simulink model "SpeedandTorqueModeComponent"  (R2026a)
settings: Solver=FixedStepDiscrete
settings Model: DataDictionary=TractionEmotorSoftwareArchInterfaceData.sldd  Creator=dakaihu  LastModifiedBy=dakaihu

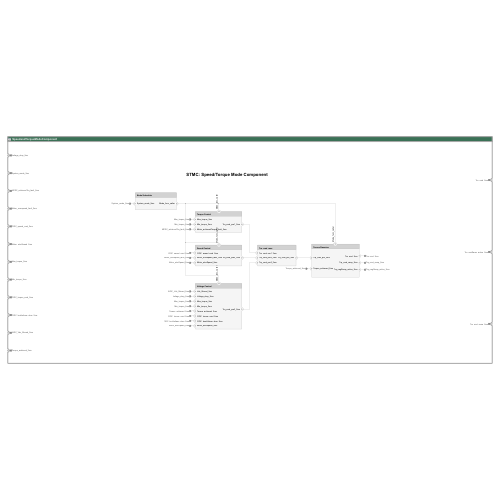
[thumbnail: Simulink's stored preview of the top-level diagram]
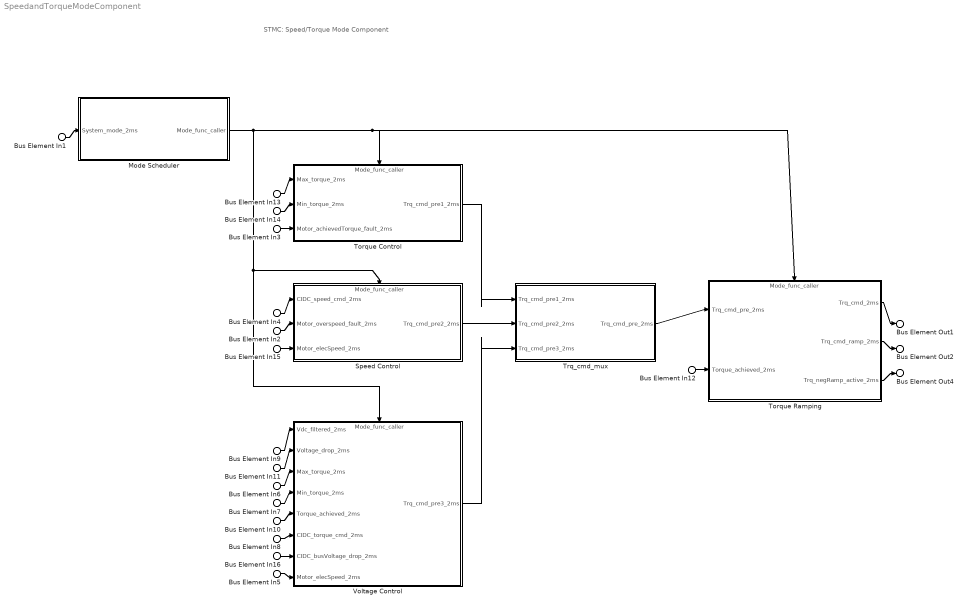
== system SpeedandTorqueModeComponent ==
  note: STMC: Speed/Torque Mode Component
  Bus Element In11 : Inport  PortName=Voltage_drop_2ms
  Bus Element In1 : Inport  Port=2  PortName=System_mode_2ms
  Bus Element In3 : Inport  Port=3  PortName=MFDC_achievedTrq_fault_2ms
  Bus Element In2 : Inport  Port=4  PortName=Motor_overspeed_fault_2ms
  Bus Element In4 : Inport  Port=5  PortName=CIDC_speed_cmd_2ms
  Bus Element In5 : Inport  Port=6  PortName=Motor_elecSpeed_2ms
  Bus Element In15 : Inport  Port=6  PortName=Motor_elecSpeed_2ms
  Bus Element In6 : Inport  Port=7  PortName=Max_torque_2ms
  Bus Element In13 : Inport  Port=7  PortName=Max_torque_2ms
  Bus Element In7 : Inport  Port=8  PortName=Min_torque_2ms
  Bus Element In14 : Inport  Port=8  PortName=Min_torque_2ms
  Bus Element In8 : Inport  Port=9  PortName=CIDC_torque_cmd_2ms
  Bus Element In16 : Inport  Port=10  PortName=CIDC_busVoltage_drop_2ms
  Bus Element In9 : Inport  Port=11  PortName=IHDC_Vdc_filtered_2ms
  Bus Element In10 : Inport  Port=12  PortName=Torque_achieved_2ms
  Bus Element In12 : Inport  Port=12  PortName=Torque_achieved_2ms
  Mode Scheduler : Subsystem
      settings: PortSchema="{\"entries\":[{\"content\":{\"headerSize\":26,\"margin\":15,\"minimumSpacing\":25,\"sides\":[{\"content\":{\"connectorIds\":[\"In1\"]},\"type\":\"ConnectorPlacement.EquallySpacedRectSide\",\"uuid\":\"b2f30fca-3d8e-46ee-af1d-282b22b9b844\"},{\"content\":{\"connectorIds\":[\"Out1\"],\"side\":\"RIGHT\"},\"type\":\"ConnectorPlacement.EquallySpacedRectSide\",\"uuid\":\"2d7d706d-eac4-4c73-84e8-2a36a393a616\"},{\"content\":{\"connectorIds\":[],\"side\":\"TOP\"},\"type\":\"ConnectorPlacement.EquallySpacedRectSide\",\"uuid\":\"b52ae510-b7cc-4ed0-8d34-4a095deae41b\"}]},\"type\":\"ConnectorPlacement.EquallySpacedConnector\",\"uuid\":\"1257e7cc-1858-4bc4-ab05-7b00060cf0d5\"}],\"packageUris\":[\"http://schema.mathworks.com/mf0/Connector/R2020b\"],\"version\":\"1.0\"}"
  Speed Control : Subsystem
      settings: PortSchema="{\"entries\":[{\"content\":{\"headerSize\":26,\"margin\":15,\"minimumSpacing\":25,\"sides\":[{\"content\":{\"connectorIds\":[\"In1\",\"In2\",\"In3\"]},\"type\":\"ConnectorPlacement.EquallySpacedRectSide\",\"uuid\":\"b2f30fca-3d8e-46ee-af1d-282b22b9b844\"},{\"content\":{\"connectorIds\":[\"Out1\"],\"side\":\"RIGHT\"},\"type\":\"ConnectorPlacement.EquallySpacedRectSide\",\"uuid\":\"2d7d706d-eac4-4c73-84e8-2a36a393a616\"},{\"content\":{\"connectorIds\":[\"In4\"],\"side\":\"TOP\"},\"type\":\"ConnectorPlacement.EquallySpacedRectSide\",\"uuid\":\"b52ae510-b7cc-4ed0-8d34-4a095deae41b\"}]},\"type\":\"ConnectorPlacement.EquallySpacedConnector\",\"uuid\":\"1257e7cc-1858-4bc4-ab05-7b00060cf0d5\"}],\"packageUris\":[\"http://schema.mathworks.com/mf0/Connector/R2020b\"],\"version\":\"1.0\"}"
  Torque Control : Subsystem
      settings: PortSchema="{\"entries\":[{\"content\":{\"headerSize\":26,\"margin\":15,\"minimumSpacing\":25,\"sides\":[{\"content\":{\"connectorIds\":[\"In1\",\"In2\",\"In3\"]},\"type\":\"ConnectorPlacement.EquallySpacedRectSide\",\"uuid\":\"b2f30fca-3d8e-46ee-af1d-282b22b9b844\"},{\"content\":{\"connectorIds\":[\"Out1\"],\"side\":\"RIGHT\"},\"type\":\"ConnectorPlacement.EquallySpacedRectSide\",\"uuid\":\"2d7d706d-eac4-4c73-84e8-2a36a393a616\"},{\"content\":{\"connectorIds\":[\"In4\"],\"side\":\"TOP\"},\"type\":\"ConnectorPlacement.EquallySpacedRectSide\",\"uuid\":\"b52ae510-b7cc-4ed0-8d34-4a095deae41b\"}]},\"type\":\"ConnectorPlacement.EquallySpacedConnector\",\"uuid\":\"1257e7cc-1858-4bc4-ab05-7b00060cf0d5\"}],\"packageUris\":[\"http://schema.mathworks.com/mf0/Connector/R2020b\"],\"version\":\"1.0\"}"
  Torque Ramping : Subsystem
      settings: PortSchema="{\"entries\":[{\"content\":{\"headerSize\":26,\"margin\":15,\"minimumSpacing\":25,\"sides\":[{\"content\":{\"connectorIds\":[\"In3\",\"In2\"]},\"type\":\"ConnectorPlacement.EquallySpacedRectSide\",\"uuid\":\"b2f30fca-3d8e-46ee-af1d-282b22b9b844\"},{\"content\":{\"connectorIds\":[\"Out1\",\"Out2\",\"Out3\"],\"side\":\"RIGHT\"},\"type\":\"ConnectorPlacement.EquallySpacedRectSide\",\"uuid\":\"2d7d706d-eac4-4c73-84e8-2a36a393a616\"},{\"content\":{\"connectorIds\":[\"In1\"],\"side\":\"TOP\"},\"type\":\"ConnectorPlacement.EquallySpacedRectSide\",\"uuid\":\"b52ae510-b7cc-4ed0-8d34-4a095deae41b\"}]},\"type\":\"ConnectorPlacement.EquallySpacedConnector\",\"uuid\":\"1257e7cc-1858-4bc4-ab05-7b00060cf0d5\"}],\"packageUris\":[\"http://schema.mathworks.com/mf0/Connector/R2020b\"],\"version\":\"1.0\"}"
  Trq_cmd_mux : Subsystem
      settings: PortSchema="{\"entries\":[{\"content\":{\"headerSize\":26,\"margin\":15,\"minimumSpacing\":25,\"sides\":[{\"content\":{\"connectorIds\":[\"In1\",\"In2\",\"In3\"]},\"type\":\"ConnectorPlacement.EquallySpacedRectSide\",\"uuid\":\"e09fe738-2b2d-403f-b055-60947e3a12a9\"},{\"content\":{\"connectorIds\":[\"Out1\"],\"side\":\"RIGHT\"},\"type\":\"ConnectorPlacement.EquallySpacedRectSide\",\"uuid\":\"7566e870-d5f8-4c16-9c2a-de0e46bcfc8a\"},{\"content\":{\"connectorIds\":[],\"side\":\"TOP\"},\"type\":\"ConnectorPlacement.EquallySpacedRectSide\",\"uuid\":\"baa3809f-6a8a-4fc9-b6be-968aafcdb1b7\"}]},\"type\":\"ConnectorPlacement.EquallySpacedConnector\",\"uuid\":\"274f79bf-3dc3-455f-a70a-3832140476bd\"}],\"packageUris\":[\"http://schema.mathworks.com/mf0/Connector/R2020b\"],\"version\":\"1.0\"}"
  Voltage Control : Subsystem
      settings: PortSchema="{\"entries\":[{\"content\":{\"headerSize\":26,\"margin\":15,\"minimumSpacing\":25,\"sides\":[{\"content\":{\"connectorIds\":[\"In1\",\"In3\",\"In2\",\"In4\",\"In5\",\"In6\",\"In8\",\"In7\"]},\"type\":\"ConnectorPlacement.EquallySpacedRectSide\",\"uuid\":\"b2f30fca-3d8e-46ee-af1d-282b22b9b844\"},{\"content\":{\"connectorIds\":[\"Out1\"],\"side\":\"RIGHT\"},\"type\":\"ConnectorPlacement.EquallySpacedRectSide\",\"uuid\":\"2d7d706d-eac4-4c73-84e8-2a36a393a616\"},{\"content\":{\"connectorIds\":[\"In9\"],\"side\":\"TOP\"},\"type\":\"ConnectorPlacement.EquallySpacedRectSide\",\"uuid\":\"b52ae510-b7cc-4ed0-8d34-4a095deae41b\"}]},\"type\":\"ConnectorPlacement.EquallySpacedConnector\",\"uuid\":\"1257e7cc-1858-4bc4-ab05-7b00060cf0d5\"}],\"packageUris\":[\"http://schema.mathworks.com/mf0/Connector/R2020b\"],\"version\":\"1.0\"}"
  Bus Element Out1 : Outport  PortName=Trq_cmd_2ms
  Bus Element Out4 : Outport  Port=2  PortName=Trq_negRamp_active_2ms
  Bus Element Out2 : Outport  Port=3  PortName=Trq_cmd_ramp_2ms
  wires:
  Torque Ramping/1(Trq_cmd_2ms) -> Bus Element Out1/1
  Torque Ramping/2(Trq_cmd_ramp_2ms) -> Bus Element Out2/1
  Bus Element In1/1 -> Mode Scheduler/1(System_mode_2ms)
  Mode Scheduler/1(Mode_func_caller) -> Voltage Control/9(Mode_func_caller), Speed Control/4(Mode_func_caller), Torque Control/4(Mode_func_caller), Torque Ramping/1(Mode_func_caller)
  Torque Control/1(Trq_cmd_pre1_2ms) -> Trq_cmd_mux/1(Trq_cmd_pre1_2ms)
  Speed Control/1(Trq_cmd_pre2_2ms) -> Trq_cmd_mux/2(Trq_cmd_pre2_2ms)
  Voltage Control/1(Trq_cmd_pre3_2ms) -> Trq_cmd_mux/3(Trq_cmd_pre3_2ms)
  Trq_cmd_mux/1(Trq_cmd_pre_2ms) -> Torque Ramping/3(Trq_cmd_pre_2ms)
  Bus Element In9/1 -> Voltage Control/1(Vdc_filtered_2ms)
  Bus Element In11/1 -> Voltage Control/3(Voltage_drop_2ms)
  Bus Element In6/1 -> Voltage Control/2(Max_torque_2ms)
  Bus Element In7/1 -> Voltage Control/4(Min_torque_2ms)
  Bus Element In10/1 -> Voltage Control/5(Torque_achieved_2ms)
  Bus Element In4/1 -> Speed Control/1(CIDC_speed_cmd_2ms)
  Bus Element In12/1 -> Torque Ramping/2(Torque_achieved_2ms)
  Bus Element In13/1 -> Torque Control/1(Max_torque_2ms)
  Bus Element In14/1 -> Torque Control/2(Min_torque_2ms)
  Bus Element In8/1 -> Voltage Control/6(CIDC_torque_cmd_2ms)
  Bus Element In2/1 -> Speed Control/2(Motor_overspeed_fault_2ms)
  Bus Element In5/1 -> Voltage Control/7(Motor_elecSpeed_2ms)
  Bus Element In15/1 -> Speed Control/3(Motor_elecSpeed_2ms)
  Bus Element In3/1 -> Torque Control/3(Motor_achievedTorque_fault_2ms)
  Torque Ramping/3(Trq_negRamp_active_2ms) -> Bus Element Out4/1
  Bus Element In16/1 -> Voltage Control/8(CIDC_busVoltage_drop_2ms)

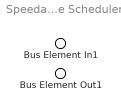
== system SpeedandTorqueModeComponent/Mode Scheduler ==
  Bus Element In1 : Inport  PortName=System_mode_2ms
  Bus Element Out1 : Outport  PortName=Mode_func_caller

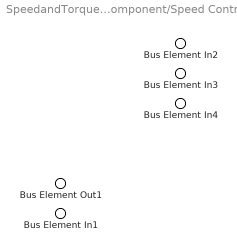
== system SpeedandTorqueModeComponent/Speed Control ==
  Bus Element In2 : Inport  PortName=CIDC_speed_cmd_2ms
  Bus Element In3 : Inport  Port=2  PortName=Motor_overspeed_fault_2ms
  Bus Element In4 : Inport  Port=3  PortName=Motor_elecSpeed_2ms
  Bus Element In1 : Inport  Port=4  PortName=Mode_func_caller
  Bus Element Out1 : Outport  PortName=Trq_cmd_pre2_2ms

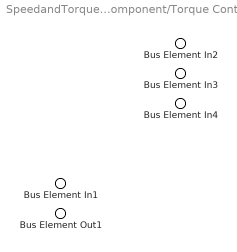
== system SpeedandTorqueModeComponent/Torque Control ==
  Bus Element In2 : Inport  PortName=Max_torque_2ms
  Bus Element In3 : Inport  Port=2  PortName=Min_torque_2ms
  Bus Element In4 : Inport  Port=3  PortName=Motor_achievedTorque_fault_2ms
  Bus Element In1 : Inport  Port=4  PortName=Mode_func_caller
  Bus Element Out1 : Outport  PortName=Trq_cmd_pre1_2ms

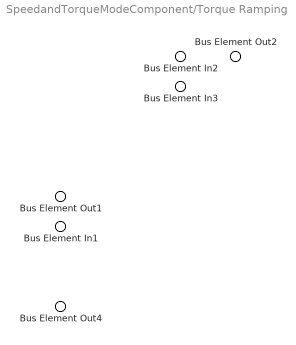
== system SpeedandTorqueModeComponent/Torque Ramping ==
  Bus Element In2 : Inport  PortName=Mode_func_caller
  Bus Element In3 : Inport  Port=2  PortName=Torque_achieved_2ms
  Bus Element In1 : Inport  Port=3  PortName=Trq_cmd_pre_2ms
  Bus Element Out2 : Outport  PortName=Trq_cmd_2ms
  Bus Element Out1 : Outport  Port=2  PortName=Trq_cmd_ramp_2ms
  Bus Element Out4 : Outport  Port=3  PortName=Trq_negRamp_active_2ms

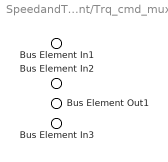
== system SpeedandTorqueModeComponent/Trq_cmd_mux ==
  Bus Element In1 : Inport  PortName=Trq_cmd_pre1_2ms
  Bus Element In2 : Inport  Port=2  PortName=Trq_cmd_pre2_2ms
  Bus Element In3 : Inport  Port=3  PortName=Trq_cmd_pre3_2ms
  Bus Element Out1 : Outport  PortName=Trq_cmd_pre_2ms

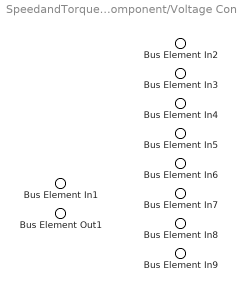
== system SpeedandTorqueModeComponent/Voltage Control ==
  Bus Element In2 : Inport  PortName=Vdc_filtered_2ms
  Bus Element In4 : Inport  Port=2  PortName=Max_torque_2ms
  Bus Element In3 : Inport  Port=3  PortName=Voltage_drop_2ms
  Bus Element In5 : Inport  Port=4  PortName=Min_torque_2ms
  Bus Element In6 : Inport  Port=5  PortName=Torque_achieved_2ms
  Bus Element In7 : Inport  Port=6  PortName=CIDC_torque_cmd_2ms
  Bus Element In8 : Inport  Port=7  PortName=Motor_elecSpeed_2ms
  Bus Element In9 : Inport  Port=8  PortName=CIDC_busVoltage_drop_2ms
  Bus Element In1 : Inport  Port=9  PortName=Mode_func_caller
  Bus Element Out1 : Outport  PortName=Trq_cmd_pre3_2ms
